simulink model "TST_PT_TrqRat"  (R2016b)
settings: Solver=FixedStepDiscrete  StartTime=0.0  StopTime=simTime  FixedStep=sampleTime  RelTol=1e-3
values from neighbouring files (symbols this model uses):
  testCase = 1    [initTST_PT_TrqRat_001.m]    (also in initTST_PT_TrqRat_002.m = 2)
libraries: simulink x7, UnitTest_Lib x4
settings Model: Creator=zhengjinyan  LastModifiedBy=zhengjinyan
settings DebuggingCC: SignalRangeChecking=error

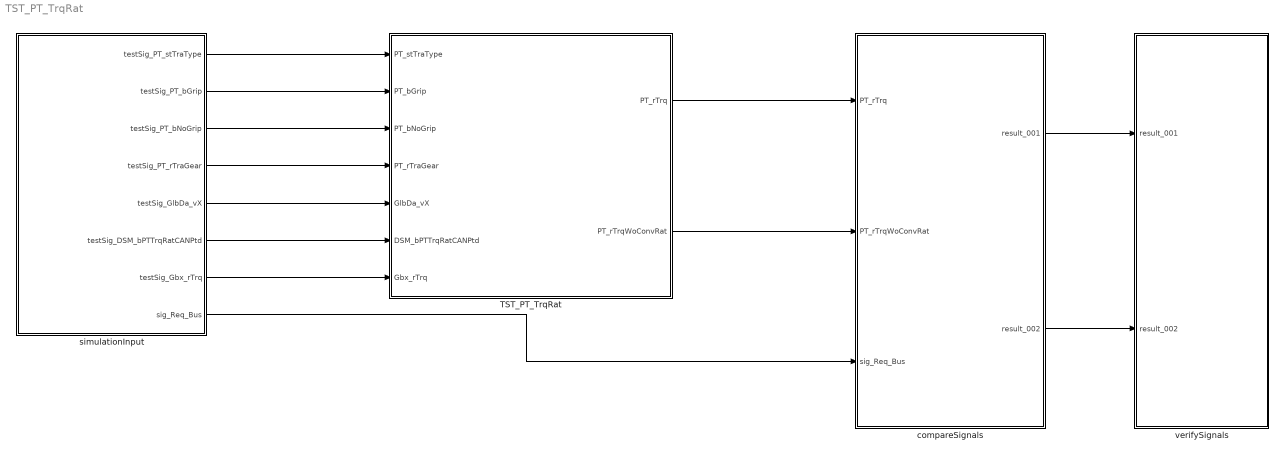
== system TST_PT_TrqRat ==
  TST_PT_TrqRat : Subsystem
  compareSignals : Subsystem
  simulationInput : Subsystem
  verifySignals : Subsystem
  wires:
  simulationInput/1(testSig_PT_stTraType) -> TST_PT_TrqRat/1(PT_stTraType)
  simulationInput/2(testSig_PT_bGrip) -> TST_PT_TrqRat/2(PT_bGrip)
  simulationInput/3(testSig_PT_bNoGrip) -> TST_PT_TrqRat/3(PT_bNoGrip)
  simulationInput/4(testSig_PT_rTraGear) -> TST_PT_TrqRat/4(PT_rTraGear)
  simulationInput/5(testSig_GlbDa_vX) -> TST_PT_TrqRat/5(GlbDa_vX)
  simulationInput/6(testSig_DSM_bPTTrqRatCANPtd) -> TST_PT_TrqRat/6(DSM_bPTTrqRatCANPtd)
  simulationInput/7(testSig_Gbx_rTrq) -> TST_PT_TrqRat/7(Gbx_rTrq)
  TST_PT_TrqRat/1(PT_rTrq) -> compareSignals/1(PT_rTrq)
  TST_PT_TrqRat/2(PT_rTrqWoConvRat) -> compareSignals/2(PT_rTrqWoConvRat)
  simulationInput/8(sig_Req_Bus) -> compareSignals/3(sig_Req_Bus)
  compareSignals/1(result_001) -> verifySignals/1(result_001)
  compareSignals/2(result_002) -> verifySignals/2(result_002)

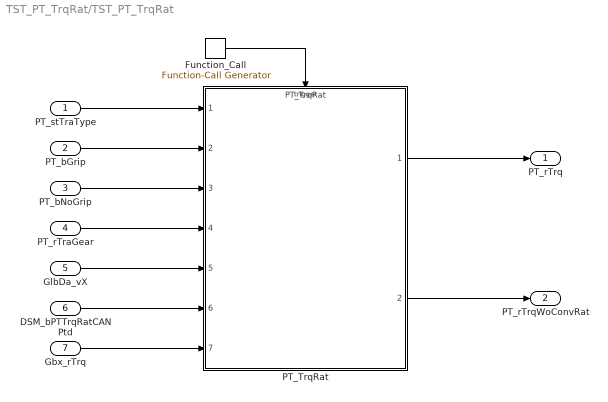
== system TST_PT_TrqRat/TST_PT_TrqRat ==
  PT_stTraType : Inport
  PT_bGrip : Inport  Port=2
  PT_bNoGrip : Inport  Port=3
  PT_rTraGear : Inport  Port=4
  GlbDa_vX : Inport  Port=5
  DSM_bPTTrqRatCANPtd : Inport  Port=6
  Gbx_rTrq : Inport  Port=7
  Function_Call : simulink/Ports & Subsystems/Function-Call Generator  sample_time=sampleTime  numberOfIterations=1
  PT_TrqRat : ModelReference  ModelNameDialog=PT_TrqRat  SimulationMode=Normal  ModelReferenceVersion=1.8  TriggerPortName=function  TriggerPortTriggerType=function-call  TriggerPortStatesWhenEnabling=held
  PT_rTrq : Outport
  PT_rTrqWoConvRat : Outport  Port=2
  wires:
  Function_Call/1 -> PT_TrqRat/Trigger
  PT_stTraType/1 -> PT_TrqRat/1
  PT_bGrip/1 -> PT_TrqRat/2
  PT_bNoGrip/1 -> PT_TrqRat/3
  PT_rTraGear/1 -> PT_TrqRat/4
  GlbDa_vX/1 -> PT_TrqRat/5
  DSM_bPTTrqRatCANPtd/1 -> PT_TrqRat/6
  Gbx_rTrq/1 -> PT_TrqRat/7
  PT_TrqRat/1 -> PT_rTrq/1
  PT_TrqRat/2 -> PT_rTrqWoConvRat/1

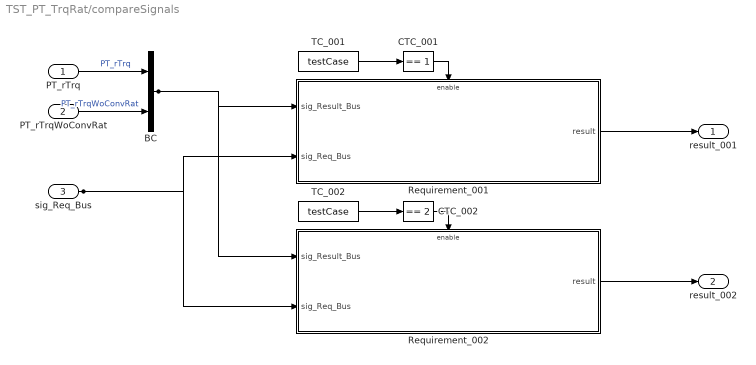
== system TST_PT_TrqRat/compareSignals ==
  PT_rTrq : Inport
  PT_rTrqWoConvRat : Inport  Port=2
  sig_Req_Bus : Inport  Port=3
  BC : BusCreator  Inputs=2
  CTC_001 : simulink/Logic and Bit Operations/Compare To Constant  relop===  const=1  OutDataTypeStr=boolean
  CTC_002 : simulink/Logic and Bit Operations/Compare To Constant  relop===  const=2  OutDataTypeStr=boolean
  Requirement_001 : Subsystem
  Requirement_002 : Subsystem
  TC_001 : Constant  Value=testCase
  TC_002 : Constant  Value=testCase
  result_001 : Outport
  result_002 : Outport  Port=2
  wires:
  PT_rTrq/1 -> BC/1  "PT_rTrq"
  PT_rTrqWoConvRat/1 -> BC/2  "PT_rTrqWoConvRat"
  TC_001/1 -> CTC_001/1
  CTC_001/1 -> Requirement_001/Enable
  sig_Req_Bus/1 -> Requirement_001/2(sig_Req_Bus), Requirement_002/2(sig_Req_Bus)
  BC/1 -> Requirement_001/1(sig_Result_Bus), Requirement_002/1(sig_Result_Bus)
  Requirement_001/1(result) -> result_001/1
  TC_002/1 -> CTC_002/1
  CTC_002/1 -> Requirement_002/Enable
  Requirement_002/1(result) -> result_002/1

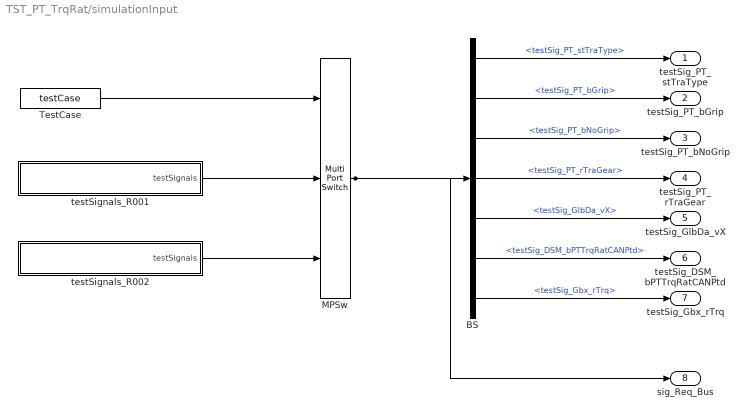
== system TST_PT_TrqRat/simulationInput ==
  BS : BusSelector  OutputSignals=testSig_PT_stTraType,testSig_PT_bGrip,testSig_PT_bNoGrip,testSig_PT_rTraGear,testSig_GlbDa_vX,testSig_DSM_bPTTrqRatCANPtd,testSig_Gbx_rTrq
  MPSw : MultiPortSwitch  Inputs=2  SaturateOnIntegerOverflow=on  InputSameDT=on
  TestCase : Constant  Value=testCase
  testSignals_R001 : Subsystem
  testSignals_R002 : Subsystem
  testSig_PT_stTraType : Outport
  testSig_PT_bGrip : Outport  Port=2
  testSig_PT_bNoGrip : Outport  Port=3
  testSig_PT_rTraGear : Outport  Port=4
  testSig_GlbDa_vX : Outport  Port=5
  testSig_DSM_bPTTrqRatCANPtd : Outport  Port=6
  testSig_Gbx_rTrq : Outport  Port=7
  sig_Req_Bus : Outport  Port=8
  wires:
  BS/1 -> testSig_PT_stTraType/1  "<testSig_PT_stTraType>"
  BS/2 -> testSig_PT_bGrip/1  "<testSig_PT_bGrip>"
  BS/3 -> testSig_PT_bNoGrip/1  "<testSig_PT_bNoGrip>"
  BS/4 -> testSig_PT_rTraGear/1  "<testSig_PT_rTraGear>"
  BS/5 -> testSig_GlbDa_vX/1  "<testSig_GlbDa_vX>"
  BS/6 -> testSig_DSM_bPTTrqRatCANPtd/1  "<testSig_DSM_bPTTrqRatCANPtd>"
  BS/7 -> testSig_Gbx_rTrq/1  "<testSig_Gbx_rTrq>"
  MPSw/1 -> BS/1, sig_Req_Bus/1
  TestCase/1 -> MPSw/1
  testSignals_R001/1(testSignals) -> MPSw/2
  testSignals_R002/1(testSignals) -> MPSw/3

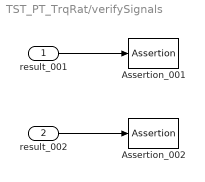
== system TST_PT_TrqRat/verifySignals ==
  result_001 : Inport
  result_002 : Inport  Port=2
  Assertion_001 : Assertion  Enabled=off
  Assertion_002 : Assertion  Enabled=off
  wires:
  result_001/1 -> Assertion_001/1
  result_002/1 -> Assertion_002/1

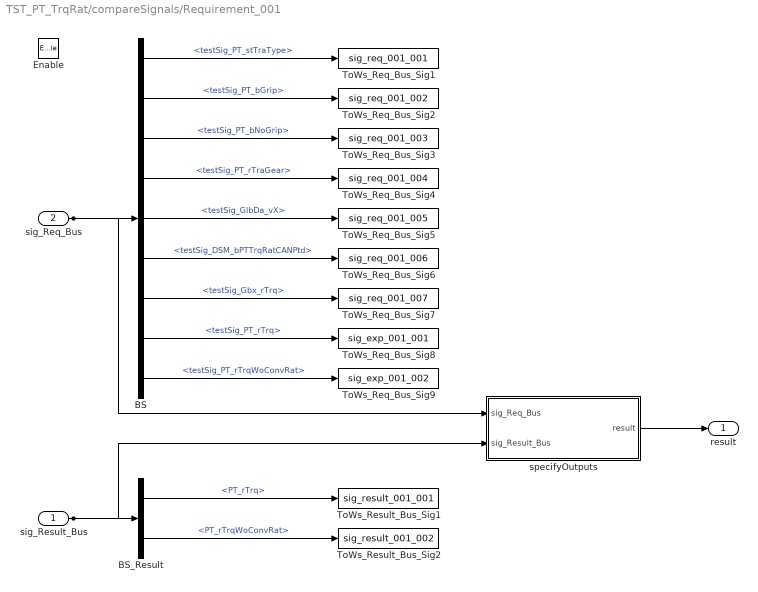
== system TST_PT_TrqRat/compareSignals/Requirement_001 ==
  sig_Result_Bus : Inport
  sig_Req_Bus : Inport  Port=2
  Enable : EnablePort
  BS : BusSelector  OutputSignals=testSig_PT_stTraType,testSig_PT_bGrip,testSig_PT_bNoGrip,testSig_PT_rTraGear,testSig_GlbDa_vX,testSig_DSM_bPTTrqRatCANPtd,testSig_Gbx_rTrq,testSig_PT_rTrq,testSig_PT_rTrqWoConvRat
  BS_Result : BusSelector  OutputSignals=PT_rTrq,PT_rTrqWoConvRat
  ToWs_Req_Bus_Sig1 : ToWorkspace  VariableName=sig_req_001_001  SaveFormat=Structure With Time
  ToWs_Req_Bus_Sig2 : ToWorkspace  VariableName=sig_req_001_002  SaveFormat=Structure With Time
  ToWs_Req_Bus_Sig3 : ToWorkspace  VariableName=sig_req_001_003  SaveFormat=Structure With Time
  ToWs_Req_Bus_Sig4 : ToWorkspace  VariableName=sig_req_001_004  SaveFormat=Structure With Time
  ToWs_Req_Bus_Sig5 : ToWorkspace  VariableName=sig_req_001_005  SaveFormat=Structure With Time
  ToWs_Req_Bus_Sig6 : ToWorkspace  VariableName=sig_req_001_006  SaveFormat=Structure With Time
  ToWs_Req_Bus_Sig7 : ToWorkspace  VariableName=sig_req_001_007  SaveFormat=Structure With Time
  ToWs_Req_Bus_Sig8 : ToWorkspace  VariableName=sig_exp_001_001  SaveFormat=Structure With Time
  ToWs_Req_Bus_Sig9 : ToWorkspace  VariableName=sig_exp_001_002  SaveFormat=Structure With Time
  ToWs_Result_Bus_Sig1 : ToWorkspace  VariableName=sig_result_001_001  SaveFormat=Structure With Time
  ToWs_Result_Bus_Sig2 : ToWorkspace  VariableName=sig_result_001_002  SaveFormat=Structure With Time
  specifyOutputs : Subsystem
  result : Outport
  wires:
  sig_Req_Bus/1 -> BS/1, specifyOutputs/1(sig_Req_Bus)
  BS/1 -> ToWs_Req_Bus_Sig1/1  "<testSig_PT_stTraType>"
  BS/2 -> ToWs_Req_Bus_Sig2/1  "<testSig_PT_bGrip>"
  BS/3 -> ToWs_Req_Bus_Sig3/1  "<testSig_PT_bNoGrip>"
  BS/4 -> ToWs_Req_Bus_Sig4/1  "<testSig_PT_rTraGear>"
  BS/5 -> ToWs_Req_Bus_Sig5/1  "<testSig_GlbDa_vX>"
  BS/6 -> ToWs_Req_Bus_Sig6/1  "<testSig_DSM_bPTTrqRatCANPtd>"
  BS/7 -> ToWs_Req_Bus_Sig7/1  "<testSig_Gbx_rTrq>"
  BS/8 -> ToWs_Req_Bus_Sig8/1  "<testSig_PT_rTrq>"
  BS/9 -> ToWs_Req_Bus_Sig9/1  "<testSig_PT_rTrqWoConvRat>"
  sig_Result_Bus/1 -> BS_Result/1, specifyOutputs/2(sig_Result_Bus)
  BS_Result/1 -> ToWs_Result_Bus_Sig1/1  "<PT_rTrq>"
  BS_Result/2 -> ToWs_Result_Bus_Sig2/1  "<PT_rTrqWoConvRat>"
  specifyOutputs/1(result) -> result/1

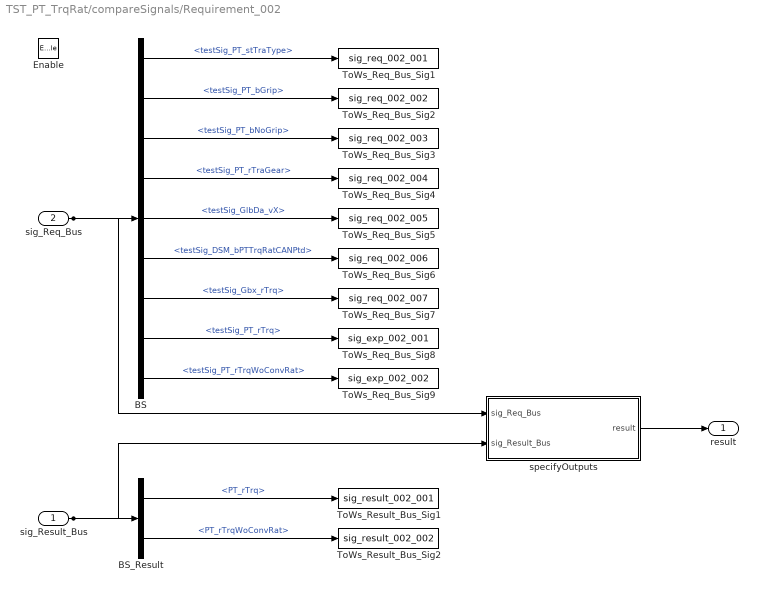
== system TST_PT_TrqRat/compareSignals/Requirement_002 ==
  sig_Result_Bus : Inport
  sig_Req_Bus : Inport  Port=2
  Enable : EnablePort
  BS : BusSelector  OutputSignals=testSig_PT_stTraType,testSig_PT_bGrip,testSig_PT_bNoGrip,testSig_PT_rTraGear,testSig_GlbDa_vX,testSig_DSM_bPTTrqRatCANPtd,testSig_Gbx_rTrq,testSig_PT_rTrq,testSig_PT_rTrqWoConvRat
  BS_Result : BusSelector  OutputSignals=PT_rTrq,PT_rTrqWoConvRat
  ToWs_Req_Bus_Sig1 : ToWorkspace  VariableName=sig_req_002_001  SaveFormat=Structure With Time
  ToWs_Req_Bus_Sig2 : ToWorkspace  VariableName=sig_req_002_002  SaveFormat=Structure With Time
  ToWs_Req_Bus_Sig3 : ToWorkspace  VariableName=sig_req_002_003  SaveFormat=Structure With Time
  ToWs_Req_Bus_Sig4 : ToWorkspace  VariableName=sig_req_002_004  SaveFormat=Structure With Time
  ToWs_Req_Bus_Sig5 : ToWorkspace  VariableName=sig_req_002_005  SaveFormat=Structure With Time
  ToWs_Req_Bus_Sig6 : ToWorkspace  VariableName=sig_req_002_006  SaveFormat=Structure With Time
  ToWs_Req_Bus_Sig7 : ToWorkspace  VariableName=sig_req_002_007  SaveFormat=Structure With Time
  ToWs_Req_Bus_Sig8 : ToWorkspace  VariableName=sig_exp_002_001  SaveFormat=Structure With Time
  ToWs_Req_Bus_Sig9 : ToWorkspace  VariableName=sig_exp_002_002  SaveFormat=Structure With Time
  ToWs_Result_Bus_Sig1 : ToWorkspace  VariableName=sig_result_002_001  SaveFormat=Structure With Time
  ToWs_Result_Bus_Sig2 : ToWorkspace  VariableName=sig_result_002_002  SaveFormat=Structure With Time
  specifyOutputs : Subsystem
  result : Outport
  wires:
  sig_Req_Bus/1 -> BS/1, specifyOutputs/1(sig_Req_Bus)
  BS/1 -> ToWs_Req_Bus_Sig1/1  "<testSig_PT_stTraType>"
  BS/2 -> ToWs_Req_Bus_Sig2/1  "<testSig_PT_bGrip>"
  BS/3 -> ToWs_Req_Bus_Sig3/1  "<testSig_PT_bNoGrip>"
  BS/4 -> ToWs_Req_Bus_Sig4/1  "<testSig_PT_rTraGear>"
  BS/5 -> ToWs_Req_Bus_Sig5/1  "<testSig_GlbDa_vX>"
  BS/6 -> ToWs_Req_Bus_Sig6/1  "<testSig_DSM_bPTTrqRatCANPtd>"
  BS/7 -> ToWs_Req_Bus_Sig7/1  "<testSig_Gbx_rTrq>"
  BS/8 -> ToWs_Req_Bus_Sig8/1  "<testSig_PT_rTrq>"
  BS/9 -> ToWs_Req_Bus_Sig9/1  "<testSig_PT_rTrqWoConvRat>"
  sig_Result_Bus/1 -> BS_Result/1, specifyOutputs/2(sig_Result_Bus)
  BS_Result/1 -> ToWs_Result_Bus_Sig1/1  "<PT_rTrq>"
  BS_Result/2 -> ToWs_Result_Bus_Sig2/1  "<PT_rTrqWoConvRat>"
  specifyOutputs/1(result) -> result/1

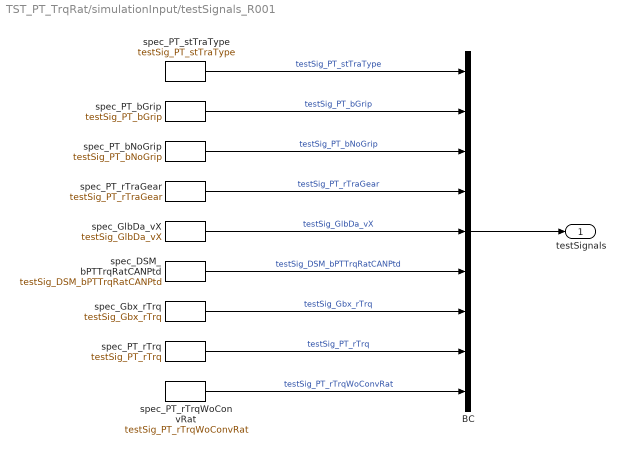
== system TST_PT_TrqRat/simulationInput/testSignals_R001 ==
  BC : BusCreator  Inputs=9
  spec_DSM_bPTTrqRatCANPtd : FromWorkspace  VariableName=testSig_DSM_bPTTrqRatCANPtd  Interpolate=off  OutputAfterFinalValue=Holding final value
  spec_Gbx_rTrq : FromWorkspace  VariableName=testSig_Gbx_rTrq  Interpolate=off  OutputAfterFinalValue=Holding final value
  spec_GlbDa_vX : FromWorkspace  VariableName=testSig_GlbDa_vX  Interpolate=off  OutputAfterFinalValue=Holding final value
  spec_PT_bGrip : FromWorkspace  VariableName=testSig_PT_bGrip  Interpolate=off  OutputAfterFinalValue=Holding final value
  spec_PT_bNoGrip : FromWorkspace  VariableName=testSig_PT_bNoGrip  Interpolate=off  OutputAfterFinalValue=Holding final value
  spec_PT_rTraGear : FromWorkspace  VariableName=testSig_PT_rTraGear  Interpolate=off  OutputAfterFinalValue=Holding final value
  spec_PT_rTrq : FromWorkspace  VariableName=testSig_PT_rTrq  Interpolate=off  OutputAfterFinalValue=Holding final value
  spec_PT_rTrqWoConvRat : FromWorkspace  VariableName=testSig_PT_rTrqWoConvRat  Interpolate=off  OutputAfterFinalValue=Holding final value
  spec_PT_stTraType : FromWorkspace  VariableName=testSig_PT_stTraType  Interpolate=off  OutputAfterFinalValue=Holding final value
  testSignals : Outport
  wires:
  BC/1 -> testSignals/1
  spec_PT_stTraType/1 -> BC/1  "testSig_PT_stTraType"
  spec_PT_bGrip/1 -> BC/2  "testSig_PT_bGrip"
  spec_PT_bNoGrip/1 -> BC/3  "testSig_PT_bNoGrip"
  spec_PT_rTraGear/1 -> BC/4  "testSig_PT_rTraGear"
  spec_GlbDa_vX/1 -> BC/5  "testSig_GlbDa_vX"
  spec_DSM_bPTTrqRatCANPtd/1 -> BC/6  "testSig_DSM_bPTTrqRatCANPtd"
  spec_Gbx_rTrq/1 -> BC/7  "testSig_Gbx_rTrq"
  spec_PT_rTrq/1 -> BC/8  "testSig_PT_rTrq"
  spec_PT_rTrqWoConvRat/1 -> BC/9  "testSig_PT_rTrqWoConvRat"

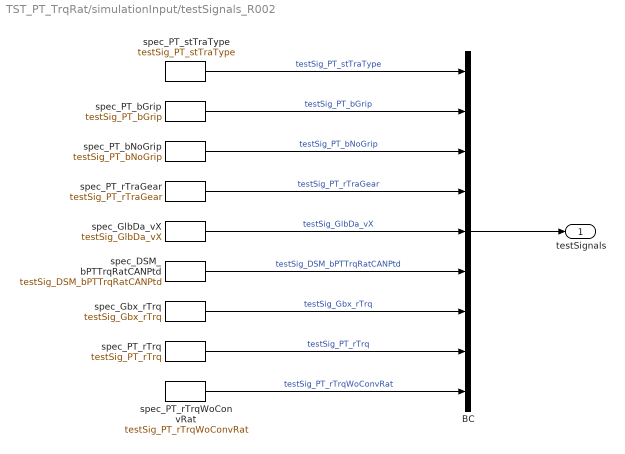
== system TST_PT_TrqRat/simulationInput/testSignals_R002 ==
  BC : BusCreator  Inputs=9
  spec_DSM_bPTTrqRatCANPtd : FromWorkspace  VariableName=testSig_DSM_bPTTrqRatCANPtd  Interpolate=off  OutputAfterFinalValue=Holding final value
  spec_Gbx_rTrq : FromWorkspace  VariableName=testSig_Gbx_rTrq  Interpolate=off  OutputAfterFinalValue=Holding final value
  spec_GlbDa_vX : FromWorkspace  VariableName=testSig_GlbDa_vX  Interpolate=off  OutputAfterFinalValue=Holding final value
  spec_PT_bGrip : FromWorkspace  VariableName=testSig_PT_bGrip  Interpolate=off  OutputAfterFinalValue=Holding final value
  spec_PT_bNoGrip : FromWorkspace  VariableName=testSig_PT_bNoGrip  Interpolate=off  OutputAfterFinalValue=Holding final value
  spec_PT_rTraGear : FromWorkspace  VariableName=testSig_PT_rTraGear  Interpolate=off  OutputAfterFinalValue=Holding final value
  spec_PT_rTrq : FromWorkspace  VariableName=testSig_PT_rTrq  Interpolate=off  OutputAfterFinalValue=Holding final value
  spec_PT_rTrqWoConvRat : FromWorkspace  VariableName=testSig_PT_rTrqWoConvRat  Interpolate=off  OutputAfterFinalValue=Holding final value
  spec_PT_stTraType : FromWorkspace  VariableName=testSig_PT_stTraType  Interpolate=off  OutputAfterFinalValue=Holding final value
  testSignals : Outport
  wires:
  BC/1 -> testSignals/1
  spec_PT_stTraType/1 -> BC/1  "testSig_PT_stTraType"
  spec_PT_bGrip/1 -> BC/2  "testSig_PT_bGrip"
  spec_PT_bNoGrip/1 -> BC/3  "testSig_PT_bNoGrip"
  spec_PT_rTraGear/1 -> BC/4  "testSig_PT_rTraGear"
  spec_GlbDa_vX/1 -> BC/5  "testSig_GlbDa_vX"
  spec_DSM_bPTTrqRatCANPtd/1 -> BC/6  "testSig_DSM_bPTTrqRatCANPtd"
  spec_Gbx_rTrq/1 -> BC/7  "testSig_Gbx_rTrq"
  spec_PT_rTrq/1 -> BC/8  "testSig_PT_rTrq"
  spec_PT_rTrqWoConvRat/1 -> BC/9  "testSig_PT_rTrqWoConvRat"

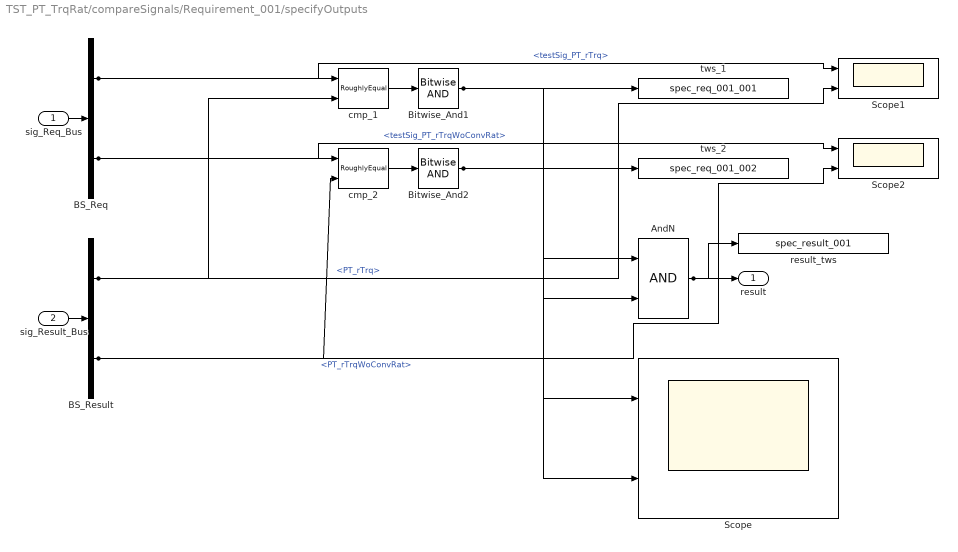
== system TST_PT_TrqRat/compareSignals/Requirement_001/specifyOutputs ==
  sig_Req_Bus : Inport
  sig_Result_Bus : Inport  Port=2
  AndN : Logic
  BS_Req : BusSelector  OutputSignals=testSig_PT_rTrq,testSig_PT_rTrqWoConvRat
  BS_Result : BusSelector  OutputSignals=PT_rTrq,PT_rTrqWoConvRat
  Bitwise_And1 : simulink/Logic and Bit Operations/Bitwise Operator  logicop=AND  UseBitMask=off  BitMask=bin2dec('11011001')  BitMaskRealWorld=Stored Integer
  Bitwise_And2 : simulink/Logic and Bit Operations/Bitwise Operator  logicop=AND  UseBitMask=off  BitMask=bin2dec('11011001')  BitMaskRealWorld=Stored Integer
  Scope : Scope  NumInputPorts=2
  Scope1 : Scope  NumInputPorts=2
  Scope2 : Scope  NumInputPorts=2
  cmp_1 : UnitTest_Lib/RoughlyEqual  slope=0.1
  cmp_2 : UnitTest_Lib/RoughlyEqual  slope=0.1
  result_tws : ToWorkspace  VariableName=spec_result_001
  tws_1 : ToWorkspace  VariableName=spec_req_001_001
  tws_2 : ToWorkspace  VariableName=spec_req_001_002
  result : Outport
  wires:
  sig_Req_Bus/1 -> BS_Req/1
  sig_Result_Bus/1 -> BS_Result/1
  AndN/1 -> result/1, result_tws/1
  BS_Req/1 -> cmp_1/1, Scope1/1  "<testSig_PT_rTrq>"
  BS_Result/1 -> cmp_1/2, Scope1/2  "<PT_rTrq>"
  cmp_1/1 -> Bitwise_And1/1
  Bitwise_And1/1 -> tws_1/1, AndN/1, Scope/1
  BS_Req/2 -> cmp_2/1, Scope2/1  "<testSig_PT_rTrqWoConvRat>"
  BS_Result/2 -> cmp_2/2, Scope2/2  "<PT_rTrqWoConvRat>"
  cmp_2/1 -> Bitwise_And2/1
  Bitwise_And2/1 -> tws_2/1, AndN/2, Scope/2

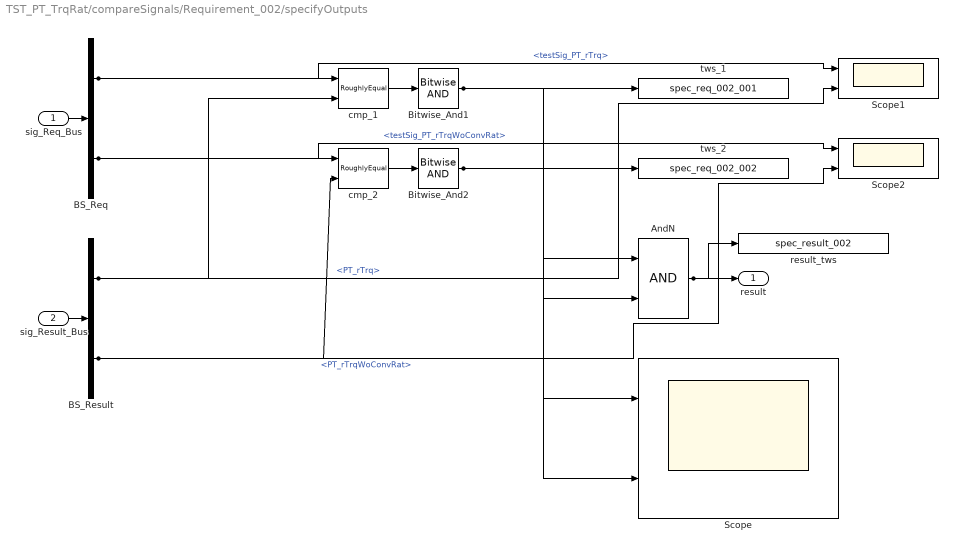
== system TST_PT_TrqRat/compareSignals/Requirement_002/specifyOutputs ==
  sig_Req_Bus : Inport
  sig_Result_Bus : Inport  Port=2
  AndN : Logic
  BS_Req : BusSelector  OutputSignals=testSig_PT_rTrq,testSig_PT_rTrqWoConvRat
  BS_Result : BusSelector  OutputSignals=PT_rTrq,PT_rTrqWoConvRat
  Bitwise_And1 : simulink/Logic and Bit Operations/Bitwise Operator  logicop=AND  UseBitMask=off  BitMask=bin2dec('11011001')  BitMaskRealWorld=Stored Integer
  Bitwise_And2 : simulink/Logic and Bit Operations/Bitwise Operator  logicop=AND  UseBitMask=off  BitMask=bin2dec('11011001')  BitMaskRealWorld=Stored Integer
  Scope : Scope  NumInputPorts=2
  Scope1 : Scope  NumInputPorts=2
  Scope2 : Scope  NumInputPorts=2
  cmp_1 : UnitTest_Lib/RoughlyEqual  slope=0.1
  cmp_2 : UnitTest_Lib/RoughlyEqual  slope=0.1
  result_tws : ToWorkspace  VariableName=spec_result_002
  tws_1 : ToWorkspace  VariableName=spec_req_002_001
  tws_2 : ToWorkspace  VariableName=spec_req_002_002
  result : Outport
  wires:
  sig_Req_Bus/1 -> BS_Req/1
  sig_Result_Bus/1 -> BS_Result/1
  AndN/1 -> result/1, result_tws/1
  BS_Req/1 -> cmp_1/1, Scope1/1  "<testSig_PT_rTrq>"
  BS_Result/1 -> cmp_1/2, Scope1/2  "<PT_rTrq>"
  cmp_1/1 -> Bitwise_And1/1
  Bitwise_And1/1 -> tws_1/1, AndN/1, Scope/1
  BS_Req/2 -> cmp_2/1, Scope2/1  "<testSig_PT_rTrqWoConvRat>"
  BS_Result/2 -> cmp_2/2, Scope2/2  "<PT_rTrqWoConvRat>"
  cmp_2/1 -> Bitwise_And2/1
  Bitwise_And2/1 -> tws_2/1, AndN/2, Scope/2
